simulink model "super"  (R2014a)
settings: Solver=ode3  StartTime=0.0  StopTime=24*3600  FixedStep=1  RelTol=1e-3
libraries: refrigeration x3
settings Model: Creator=avenger  LastModifiedBy=avenger
settings DataIOCC: LimitDataPoints=off

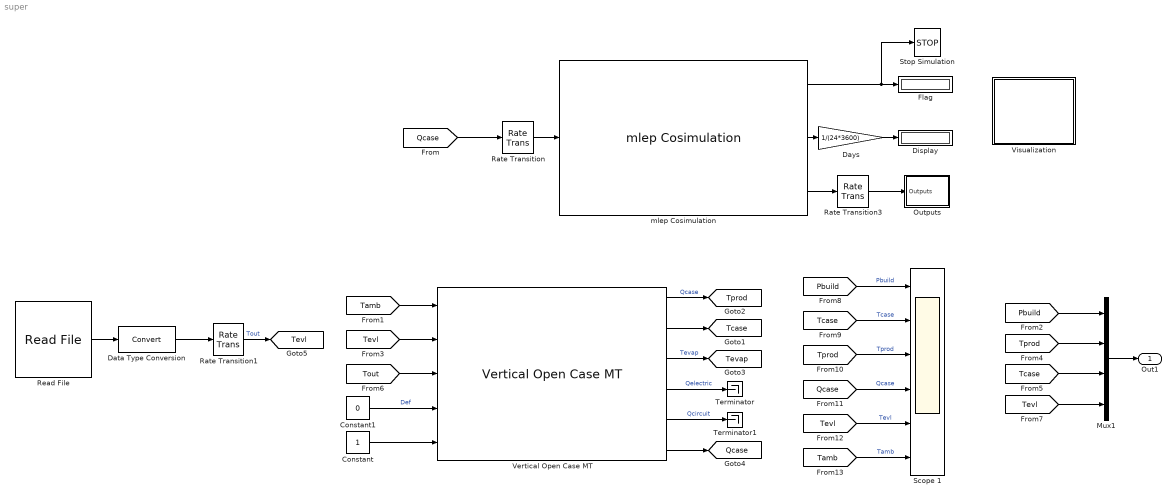
== system super ==
  Constant : Constant
  Constant1 : Constant  Value=0
  Data Type Conversion : DataTypeConversion
  Days : Gain  Gain=1/(24*3600)
  Display : Display
  Flag : Display
  Mux1 : Mux
  Outputs : Subsystem
  Rate Transition : RateTransition
  Rate Transition1 : RateTransition
  Rate Transition3 : RateTransition
  Read File : refrigeration/Read File  filename='input.txt'  timestep=3600
  Scope 1 : Scope  NumInputPorts=6
      settings: ShowLegends=on  TimeRange=90000  YMin=0~-30~-30~-20000~-30~0  YMax=200000~0~0~20000~0~20  SaveName=ScopeData2
  Stop Simulation : Stop
  Terminator : Terminator
  Terminator1 : Terminator
  Vertical Open Case MT : refrigeration/Vertical Open Case MT
  Visualization : Subsystem
  mlep Cosimulation : refrigeration/mlep Cosimulation  progname='runenergyplus'  idf='supermarket_V810'  weather='USA_FL_Miami.Intl.AP.722020_TMY3'  timeout=2000  step=300  numinput=1  numoutput=12  bcvtbpath='/home/avenger/Documents/Git/mlep_v2.0/MLE+/bcvtb'
  Out1 : Outport  InitialOutput=0
  tag scope: Qcase=global, Tcase=global, Tevap=global, Tevl=global, Tprod=global
  wires:
  [Tevl] -> Vertical Open Case MT/2
  Constant/1 -> Vertical Open Case MT/5
  Constant1/1 -> Vertical Open Case MT/4  "Def"
  Vertical Open Case MT/6 -> [Qcase]
  [Tamb] -> Vertical Open Case MT/1
  [Tout] -> Vertical Open Case MT/3
  mlep Cosimulation/2 -> Days/1
  mlep Cosimulation/1 -> Stop Simulation/1, Flag/1
  mlep Cosimulation/3 -> Rate Transition3/1
  Days/1 -> Display/1
  Rate Transition3/1 -> Outputs/1(Outputs)
  [Qcase] -> Rate Transition/1
  Rate Transition/1 -> mlep Cosimulation/1
  [Tprod] -> Mux1/2
  [Tcase] -> Mux1/3
  Mux1/1 -> Out1/1
  [Pbuild] -> Mux1/1
  Read File/1 -> Data Type Conversion/1
  Data Type Conversion/1 -> Rate Transition1/1
  Rate Transition1/1 -> [Tevl]  "Tout"
  [Tevl] -> Mux1/4
  Vertical Open Case MT/1 -> [Tprod]  "Qcase"
  Vertical Open Case MT/2 -> [Tcase]
  Vertical Open Case MT/3 -> [Tevap]  "Tevap"
  Vertical Open Case MT/4 -> Terminator/1  "Qelectric"
  Vertical Open Case MT/5 -> Terminator1/1  "Qcircuit"
  [Pbuild] -> Scope 1/1  "Pbuild"
  [Tcase] -> Scope 1/2  "Tcase"
  [Tprod] -> Scope 1/3  "Tprod"
  [Qcase] -> Scope 1/4  "Qcase"
  [Tevl] -> Scope 1/5  "Tevl"
  [Tamb] -> Scope 1/6  "Tamb"

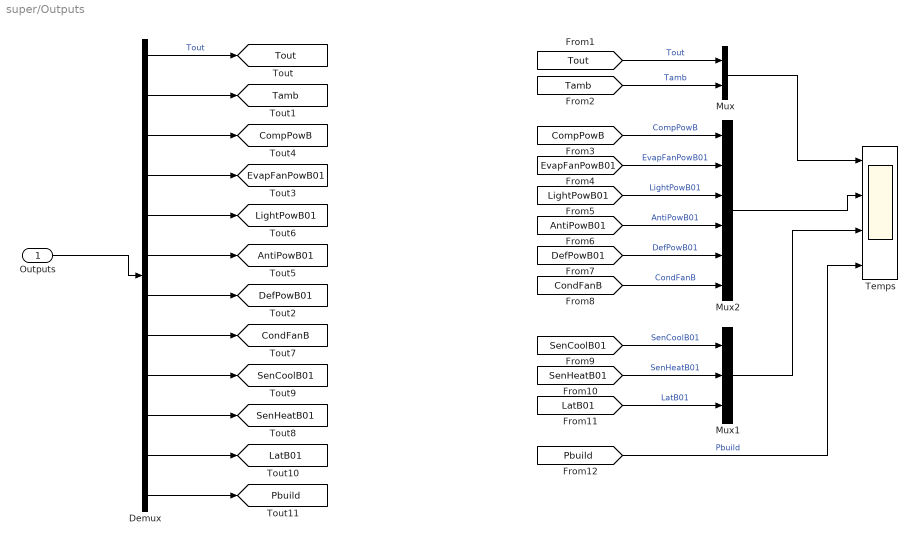
== system super/Outputs ==
  Outputs : Inport
  Demux : Demux  Outputs=12
  Mux : Mux  Inputs=2
  Mux1 : Mux  Inputs=3
  Mux2 : Mux  Inputs=6
  Temps : Scope  NumInputPorts=4
      settings: ShowLegends=on  TimeRange=90000  YMin=0~0~-500~0  YMax=35~14000~2000~200000
  tag scope: AntiPowB01=global, CompPowB=global, CondFanB=global, DefPowB01=global, EvapFanPowB01=global, LatB01=global, LightPowB01=global, Pbuild=global, SenCoolB01=global, SenHeatB01=global, Tamb=global, Tout=global
  wires:
  Outputs/1 -> Demux/1
  Demux/1 -> [Tout]  "Tout"
  Demux/2 -> [Tamb]
  Demux/3 -> [CompPowB]
  Demux/4 -> [EvapFanPowB01]
  Demux/5 -> [LightPowB01]
  Demux/6 -> [AntiPowB01]
  Demux/7 -> [DefPowB01]
  [Tout] -> Mux/1  "Tout"
  [Tamb] -> Mux/2  "Tamb"
  [CompPowB] -> Mux2/1  "CompPowB"
  [EvapFanPowB01] -> Mux2/2  "EvapFanPowB01"
  Mux2/1 -> Temps/2
  [AntiPowB01] -> Mux2/4  "AntiPowB01"
  [LightPowB01] -> Mux2/3  "LightPowB01"
  [DefPowB01] -> Mux2/5  "DefPowB01"
  Demux/8 -> [CondFanB]
  [CondFanB] -> Mux2/6  "CondFanB"
  Demux/9 -> [SenCoolB01]
  Demux/10 -> [SenHeatB01]
  Demux/11 -> [LatB01]
  Mux1/1 -> Temps/3
  [SenCoolB01] -> Mux1/1  "SenCoolB01"
  [SenHeatB01] -> Mux1/2  "SenHeatB01"
  [LatB01] -> Mux1/3  "LatB01"
  Mux/1 -> Temps/1
  Demux/12 -> [Pbuild]
  [Pbuild] -> Temps/4  "Pbuild"

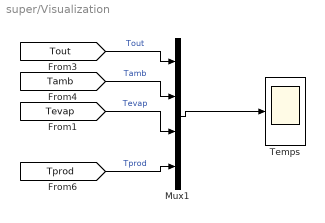
== system super/Visualization ==
  Mux1 : Mux
  Temps : Scope
      settings: ShowLegends=on  TimeRange=90000  YMin=-40  YMax=40
  wires:
  Mux1/1 -> Temps/1
  [Tout] -> Mux1/1  "Tout"
  [Tamb] -> Mux1/2  "Tamb"
  [Tevap] -> Mux1/3  "Tevap"
  [Tprod] -> Mux1/4  "Tprod"
